simulink model "DSTATCOM"  (R2023b)
settings: Solver=ode5  StartTime=0.0  StopTime=1  FixedStep=50e-8  RelTol=1e-3
InitFcn:
  | v= 400
  | p= 2500
  | q=1500
  | s=2915.47
undefined symbols (not defined in the file): DiscIntNeverNeededParam
libraries: spsThreePhaseVIMeasurementLib x11, spsThreePhaseSeriesRLCBranchLib x9, spsThreePhaseSeriesRLCLoadLib x8, spsSeriesRLCBranchLib x6, spsSecondOrderFilterLib x4, slpidlib x4, spsGroundLib x3, spsLinearTransformerLib x3, spsRMSLib x3, spsUniversalBridgeLib x2, spsabctodq0Lib x2, spsPWMGenerator2LevelLib x2
(part 1 of 2)
settings Model: Creator=prabh  LastModifiedBy=Sandesh

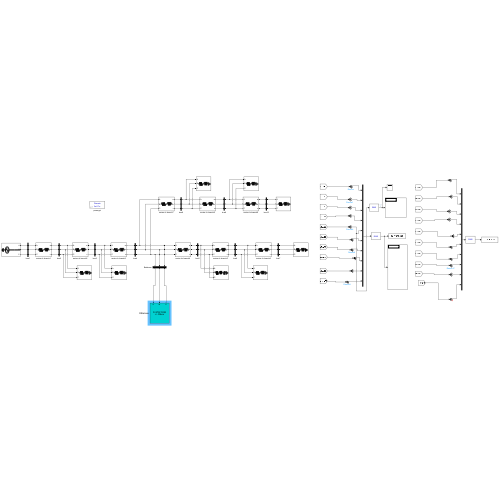
[thumbnail: Simulink's stored preview of the top-level diagram]
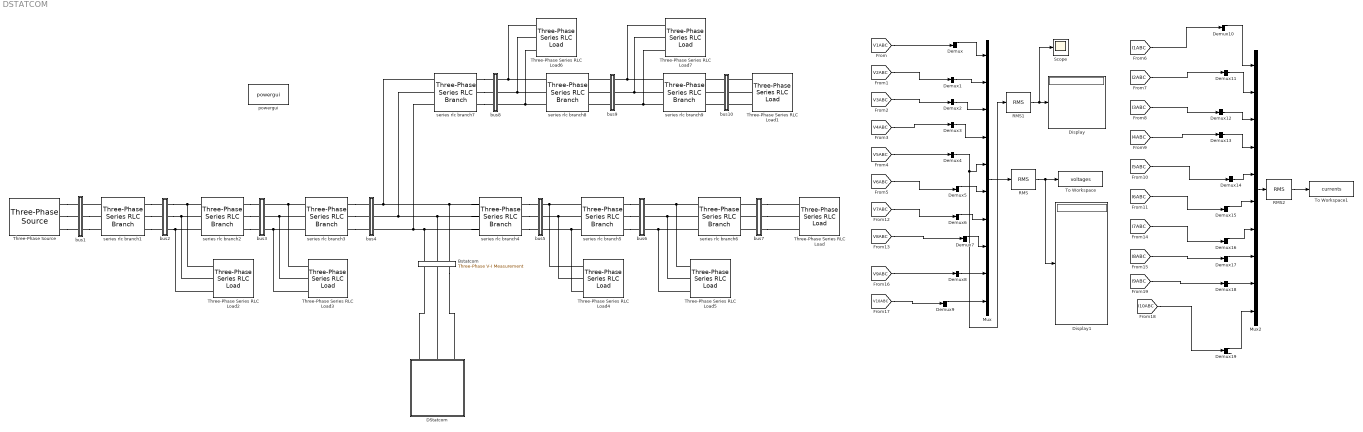
== system DSTATCOM ==
  Bstatcom : spsThreePhaseVIMeasurementLib/Three-Phase V-I Measurement  VoltageMeasurement=phase-to-ground  SetLabelV=on  LabelV=Vabc_Bstatcom  Vpu=on  VpuLL=off  CurrentMeasurement=yes  SetLabelI=on  LabelI=Iabc_Bstatcom  Ipu=on  Pbase=3e3  Vbase=400  OutputType=Magnitude  PhasorSimulation=off  PSBequivalent=0
  DStatcom : Subsystem
      mask Display: disp('D-STATCOM\n+/- 3Mvar')
  Demux{,1..19} (20 alike) : Demux  Outputs=3
  Display : Display
  Display1 : Display
  Mux : Mux  Inputs=10
  Mux2 : Mux  Inputs=10
  RMS : spsRMSLib/RMS  TrueRMS=on  Freq=50  RMSInit=0  Ts=0
  RMS1 : spsRMSLib/RMS  TrueRMS=on  Freq=50  RMSInit=0  Ts=0
  RMS2 : spsRMSLib/RMS  TrueRMS=on  Freq=50  RMSInit=0  Ts=0
  Scope : Scope
  Three-Phase Series RLC Load{,1..3,5..7} (7 alike) : spsThreePhaseSeriesRLCLoadLib/Three-Phase Series RLC Load  LConnTagsString=A|B|C  Configuration=Y (grounded)  NominalVoltage=v  Vabc=[1e3 1e3 1e3]  Vabcp=[1e3 1e3 1e3]  NominalFrequency=50  UnbalancedPower=off  ActivePower=p  InductivePower=q  CapacitivePower=0  Pabc=[10e3 9e3 11e3]  QLabc=[100 90 110]  QCabc=[100 90 110]  Pabcp=[10e3 9e3 11e3]  QLabcp=[100 90 110]  QCabcp=[100 90 110]  Measurements=None  LoadType=constant PQ
  Three-Phase Series RLC Load4 : spsThreePhaseSeriesRLCLoadLib/Three-Phase Series RLC Load  LConnTagsString=A|B|C  Configuration=Y (grounded)  NominalVoltage=v  Vabc=[1e3 1e3 1e3]  Vabcp=[1e3 1e3 1e3]  NominalFrequency=50  UnbalancedPower=off  ActivePower=p  InductivePower=q  CapacitivePower=q  Pabc=[10e3 9e3 11e3]  QLabc=[100 90 110]  QCabc=[100 90 110]  Pabcp=[10e3 9e3 11e3]  QLabcp=[100 90 110]  QCabcp=[100 90 110]  Measurements=None  LoadType=constant PQ
  Three-Phase Source : spsThreePhaseSourceLib/Three-Phase Source  InternalConnection=Yg  VoltagePhases=off  Voltage=400  PhaseAngle=0  Voltage_phases=[25e3 25e3 25e3]/sqrt(3)  PhaseAngles_phases=[0 -120 +120]  Frequency=50  NonIdealSource=off  SpecifyImpedance=off  Resistance=0.8929  Inductance=16.58e-3  ShortCircuitLevel=100e6  BaseVoltage=25e3  XRratio=7  BusType=swing  Pref=10e3  Qref=0  Prefabc=[10e3, 10e3, 10e3]  Qrefabc=[0, 0, 0]  Qmin=-inf  Qmax=inf
  To Workspace : ToWorkspace  VariableName=voltages  SampleTime=-1
      settings: MaxDataPoints=1
  To Workspace1 : ToWorkspace  VariableName=currents  SampleTime=-1
      settings: MaxDataPoints=1
  bus1 : Subsystem
  bus10 : Subsystem
  bus2 : Subsystem
  bus3 : Subsystem
  bus4 : Subsystem
  bus5 : Subsystem
  bus6 : Subsystem
  bus7 : Subsystem
  bus8 : Subsystem
  bus9 : Subsystem
  powergui : sps_lib/powergui  Priority=1  SimulationMode=Discrete  SampleTime=50e-8  frequency=60  Iterations=50  frequencyindice=50  Pbase=100e6  ErrMax=1e-4  UnitsV=kV  UnitsW=MW  buscounter=0  FunctionMessages=off  echomessages=off  EnableUseOfTLC=off  CurrentSourceSwitches=off  DisableSnubberDevices=off  DisableRonSwitches=off  DisableVfSwitches=off  DisplayEquations=off  AutomaticDiscreteSolvers=off  SolverType=Tustin/Backward Euler (TBE)  Interpol=off  ExternalGateDelay=off  methode=off  Ts=100  x0status=blocks  SPID=on  SwTol=0  HookPort=off  NonlinearTolerance=1e-4  nMaxIteration=100  ContinueOnMaxIteration=off  RestoreLinks=warning  ResistiveCurrentMeasurement=off  Frange=[0:2:500]  Ylog=off  Xlog=on  ShowGrid=off  save=off  variable=ZData  structure=0  ZoomFFT=off  StartTime=0.0  cycles=1  DisplayStyle=1  fundamental=60  FreqAxis=off  MaxFrequency=1000  frequencyindicesteady=1  RmsSteady=1  display=off
  series rlc branch1 : spsThreePhaseSeriesRLCBranchLib/Three-Phase Series RLC Branch  LConnTagsString=A|B|C  RConnTagsString=A|B|C  BranchType=RL  Resistance=0.12  Inductance=0.00027  Capacitance=0  Measurements=None
  series rlc branch2 : spsThreePhaseSeriesRLCBranchLib/Three-Phase Series RLC Branch  LConnTagsString=A|B|C  RConnTagsString=A|B|C  BranchType=RL  Resistance=.78  Inductance=.00177  Capacitance=0  Measurements=None
  series rlc branch3 : spsThreePhaseSeriesRLCBranchLib/Three-Phase Series RLC Branch  LConnTagsString=A|B|C  RConnTagsString=A|B|C  BranchType=RL  Resistance=.96  Inductance=.00218  Capacitance=0  Measurements=None
  series rlc branch4 : spsThreePhaseSeriesRLCBranchLib/Three-Phase Series RLC Branch  LConnTagsString=A|B|C  RConnTagsString=A|B|C  BranchType=RL  Resistance=.96  Inductance=.00218  Capacitance=0  Measurements=None
  series rlc branch5 : spsThreePhaseSeriesRLCBranchLib/Three-Phase Series RLC Branch  LConnTagsString=A|B|C  RConnTagsString=A|B|C  BranchType=RL  Resistance=.36  Inductance=.000821  Capacitance=0  Measurements=None
  series rlc branch6 : spsThreePhaseSeriesRLCBranchLib/Three-Phase Series RLC Branch  LConnTagsString=A|B|C  RConnTagsString=A|B|C  BranchType=RL  Resistance=.3  Inductance=.00068  Capacitance=0  Measurements=None
  series rlc branch7 : spsThreePhaseSeriesRLCBranchLib/Three-Phase Series RLC Branch  LConnTagsString=A|B|C  RConnTagsString=A|B|C  BranchType=RL  Resistance=.18  Inductance=.00041  Capacitance=0  Measurements=None
  series rlc branch8 : spsThreePhaseSeriesRLCBranchLib/Three-Phase Series RLC Branch  LConnTagsString=A|B|C  RConnTagsString=A|B|C  BranchType=RL  Resistance=.12  Inductance=.00027  Capacitance=0  Measurements=None
  series rlc branch9 : spsThreePhaseSeriesRLCBranchLib/Three-Phase Series RLC Branch  LConnTagsString=A|B|C  RConnTagsString=A|B|C  BranchType=RL  Resistance=.6  Inductance=.00136  Capacitance=0  Measurements=None
  wires:
  Mux/1 -> RMS/1
  [V1ABC] -> Demux/1
  Demux/1 -> Mux/1
  [V10ABC] -> Demux9/1
  [V9ABC] -> Demux8/1
  [V8ABC] -> Demux7/1
  [V7ABC] -> Demux6/1
  [V6ABC] -> Demux5/1
  [V5ABC] -> Demux4/1
  [V4ABC] -> Demux3/1
  [V3ABC] -> Demux2/1
  [V2ABC] -> Demux1/1
  Demux1/2 -> Mux/2
  Demux2/2 -> Mux/3
  Demux3/2 -> Mux/4
  Demux4/2 -> RMS1/1, Mux/5
  Demux5/1 -> Mux/6
  Demux6/1 -> Mux/7
  Demux7/1 -> Mux/8
  Demux8/2 -> Mux/9
  Demux9/1 -> Mux/10
  [I3ABC] -> Demux12/1
  Demux19/3 -> ?
  [I8ABC] -> Demux17/1
  [I9ABC] -> Demux18/1
  [I10ABC] -> Demux19/1
  [I4ABC] -> Demux13/1
  Demux11/2 -> Mux2/2
  Demux12/2 -> Mux2/3
  Demux18/2 -> Mux2/9
  Demux19/1 -> Mux2/10
  [I6ABC] -> Demux15/1
  [I7ABC] -> Demux16/1
  [I1ABC] -> Demux10/1
  Demux10/1 -> Mux2/1
  Demux13/2 -> Mux2/4
  Demux16/1 -> Mux2/7
  Demux15/1 -> Mux2/6
  Demux14/2 -> Mux2/5
  [I5ABC] -> Demux14/1
  Mux2/1 -> RMS2/1
  [I2ABC] -> Demux11/1
  Demux17/1 -> Mux2/8
  RMS/1 -> Display1/1, To Workspace/1
  RMS2/1 -> To Workspace1/1
  RMS1/1 -> Scope/1, Display/1
  connections:
  series rlc branch1/LConn1 -- bus1/RConn1
  bus1/RConn2 -- series rlc branch1/LConn2
  bus1/RConn3 -- series rlc branch1/LConn3
  Three-Phase Source/RConn2 -- bus1/LConn2
  Three-Phase Source/RConn1 -- bus1/LConn1
  Three-Phase Source/RConn3 -- bus1/LConn3
  series rlc branch1/RConn2 -- bus2/LConn2
  series rlc branch1/RConn1 -- bus2/LConn1
  series rlc branch1/RConn3 -- bus2/LConn3
  series rlc branch2/RConn2 -- bus3/LConn2
  series rlc branch3/LConn2 -- Three-Phase Series RLC Load3/LConn2 -- bus3/RConn2
  bus2/RConn1 -- Three-Phase Series RLC Load2/LConn1 -- series rlc branch2/LConn1
  series rlc branch2/RConn1 -- bus3/LConn1
  series rlc branch2/RConn3 -- bus3/LConn3
  series rlc branch3/LConn1 -- Three-Phase Series RLC Load3/LConn1 -- bus3/RConn1
  bus2/RConn2 -- Three-Phase Series RLC Load2/LConn2 -- series rlc branch2/LConn2
  bus2/RConn3 -- Three-Phase Series RLC Load2/LConn3 -- series rlc branch2/LConn3
  series rlc branch3/LConn3 -- Three-Phase Series RLC Load3/LConn3 -- bus3/RConn3
  series rlc branch3/RConn2 -- bus4/LConn2
  series rlc branch4/LConn2 -- Bstatcom/LConn2 -- bus4/RConn2 -- series rlc branch7/LConn2
  series rlc branch3/RConn1 -- bus4/LConn1
  series rlc branch3/RConn3 -- bus4/LConn3
  series rlc branch4/LConn1 -- Bstatcom/LConn3 -- series rlc branch7/LConn1 -- bus4/RConn1
  series rlc branch4/LConn3 -- Bstatcom/LConn1 -- bus4/RConn3 -- series rlc branch7/LConn3
  series rlc branch4/RConn2 -- bus5/LConn2
  series rlc branch5/LConn2 -- Three-Phase Series RLC Load4/LConn2 -- bus5/RConn2
  series rlc branch4/RConn1 -- bus5/LConn1
  series rlc branch4/RConn3 -- bus5/LConn3
  series rlc branch5/LConn1 -- Three-Phase Series RLC Load4/LConn1 -- bus5/RConn1
  series rlc branch5/LConn3 -- bus5/RConn3 -- Three-Phase Series RLC Load4/LConn3
  series rlc branch5/RConn2 -- bus6/LConn2
  series rlc branch6/LConn2 -- Three-Phase Series RLC Load5/LConn2 -- bus6/RConn2
  series rlc branch5/RConn1 -- bus6/LConn1
  series rlc branch5/RConn3 -- bus6/LConn3
  series rlc branch6/LConn1 -- Three-Phase Series RLC Load5/LConn1 -- bus6/RConn1
  series rlc branch6/LConn3 -- Three-Phase Series RLC Load5/LConn3 -- bus6/RConn3
  series rlc branch8/LConn3 -- Three-Phase Series RLC Load6/LConn3 -- bus8/RConn3
  series rlc branch8/LConn2 -- Three-Phase Series RLC Load6/LConn2 -- bus8/RConn2
  series rlc branch8/LConn1 -- Three-Phase Series RLC Load6/LConn1 -- bus8/RConn1
  series rlc branch7/RConn1 -- bus8/LConn1
  series rlc branch7/RConn2 -- bus8/LConn2
  series rlc branch7/RConn3 -- bus8/LConn3
  bus7/LConn1 -- series rlc branch6/RConn1
  bus7/LConn2 -- series rlc branch6/RConn2
  bus7/LConn3 -- series rlc branch6/RConn3
  bus7/RConn1 -- Three-Phase Series RLC Load/LConn1
  bus7/RConn2 -- Three-Phase Series RLC Load/LConn2
  bus7/RConn3 -- Three-Phase Series RLC Load/LConn3
  bus9/LConn1 -- series rlc branch8/RConn1
  bus9/LConn2 -- series rlc branch8/RConn2
  bus9/LConn3 -- series rlc branch8/RConn3
  series rlc branch9/LConn1 -- Three-Phase Series RLC Load7/LConn1 -- bus9/RConn1
  series rlc branch9/LConn2 -- Three-Phase Series RLC Load7/LConn2 -- bus9/RConn2
  series rlc branch9/LConn3 -- Three-Phase Series RLC Load7/LConn3 -- bus9/RConn3
  bus10/LConn1 -- series rlc branch9/RConn1
  bus10/LConn2 -- series rlc branch9/RConn2
  bus10/LConn3 -- series rlc branch9/RConn3
  Three-Phase Series RLC Load1/LConn1 -- bus10/RConn1
  Three-Phase Series RLC Load1/LConn2 -- bus10/RConn2
  Three-Phase Series RLC Load1/LConn3 -- bus10/RConn3
  DStatcom/RConn1 -- Bstatcom/RConn1
  Bstatcom/RConn3 -- DStatcom/RConn3
  DStatcom/RConn2 -- Bstatcom/RConn2

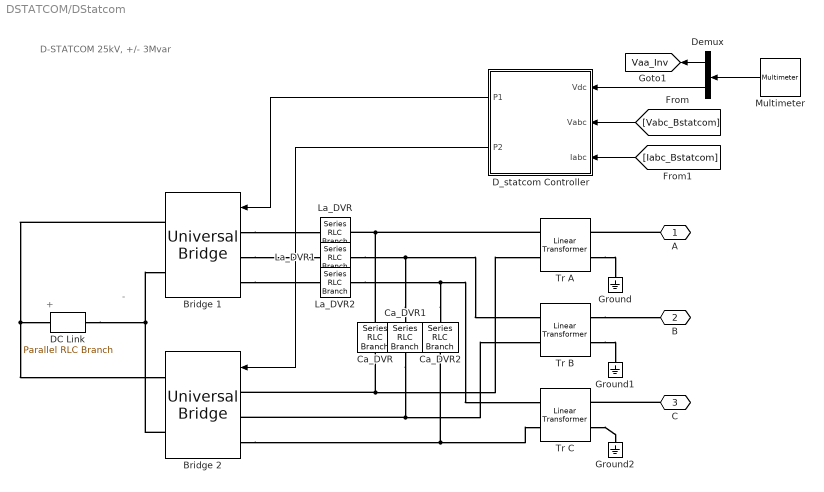
== system DSTATCOM/DStatcom ==
  note: +
  note: -
  note: D-STATCOM
      | 25kV, +/- 3Mvar
  "Bridge 1 " : spsUniversalBridgeLib/Universal Bridge  Arms=3  SnubberResistance=1e5  SnubberCapacitance=inf  Device=IGBT / Diodes  Ron=1e-3  Lon=0  ForwardVoltages="[  2  0.8  ]"  ForwardVoltage=.8  GTOparameters=[ 10e-6 , 20e-6 ]  IGBTparameters=[ 0 0]  Measurements=Device voltages  Measurements_2=None  converterType=Rectifier
      settings: AttributesFormatString=\n
  Bridge 2 : spsUniversalBridgeLib/Universal Bridge  Arms=3  SnubberResistance=1e5  SnubberCapacitance=inf  Device=IGBT / Diodes  Ron=1e-3  Lon=0  ForwardVoltages="[  2  0.8  ]"  ForwardVoltage=.8  GTOparameters=[ 10e-6 , 20e-6 ]  IGBTparameters=[ 0 0]  Measurements=Device voltages  Measurements_2=None  converterType=Rectifier
      settings: AttributesFormatString=\n
  Ca_DVR : spsSeriesRLCBranchLib/Series RLC Branch  LConnTagsString=__new0  RConnTagsString=__new0  BranchType=RC  Resistance=100e-6*(2*pi*60)/40  Inductance=1.0  SetiL0=off  InitialCurrent=0  Capacitance=100e-6  Setx0=off  InitialVoltage=0  Measurements=None
  Ca_DVR1 : spsSeriesRLCBranchLib/Series RLC Branch  LConnTagsString=__new0  RConnTagsString=__new0  BranchType=RC  Resistance=100e-6*(2*pi*60)/40  Inductance=1.0  SetiL0=off  InitialCurrent=0  Capacitance=100e-6  Setx0=off  InitialVoltage=0  Measurements=None
  Ca_DVR2 : spsSeriesRLCBranchLib/Series RLC Branch  LConnTagsString=__new0  RConnTagsString=__new0  BranchType=RC  Resistance=100e-6*(2*pi*60)/40  Inductance=1.0  SetiL0=off  InitialCurrent=0  Capacitance=100e-6  Setx0=off  InitialVoltage=0  Measurements=None
  DC Link : spsParallelRLCBranchLib/Parallel RLC Branch  LConnTagsString=a  RConnTagsString=__new0  BranchType=C  Resistance=1.0  Inductance=1.0  SetiL0=off  InitialCurrent=0  Capacitance=5000e-6  Setx0=on  InitialVoltage=0  Measurements=Branch voltage
  D_statcom Controller : Subsystem  mask(D-STATCOM Controller){ModeOper=Voltage regulation, Vac_Ref=1.0, Qref=0, Vdc_Ref=2400, Par_VacReg=[0.55 2500], Par_VdcReg=[0.001 0.15], Par_IReg=[0.8 200 0], Ts=50e-8}
      mask prompts: ModeOper "Mode of operation:"; Vac_Ref "AC voltage setpoint Vref (pu):"; Qref "Manual mode: Qref (Reactive power in pu):"; Vdc_Ref "DC Voltage setpoint (Volts)"; Par_VacReg "Vac Regulator Gains: [ Kp  Ki ]"; Par_VdcReg "Vdc Regulator Gains: [ Kp  Ki ]"; Par_IReg "Current Regulators Gain: [ Kp Ki Kd ]"; Ts "Sample time (s)"
      mask init:
      | Kp_I=Par_IReg(1);
      | Ki_I=Par_IReg(2);
      | Kd_I=Par_IReg(3);
      | Kp_Vdc=Par_VdcReg(1);
      | Ki_Vdc=Par_VdcReg(2);
      | Kp_Vac=Par_VacReg(1);
      | Ki_Vac=Par_VacReg(2);
      mask TypeOptions ModeOper: Voltage regulation | Q regulation
  Demux : Demux  Outputs=[2 1 ]
      settings: DisplayOption=none
  Ground : spsGroundLib/Ground  LConnTagsString=a
  Ground1 : spsGroundLib/Ground  LConnTagsString=a
  Ground2 : spsGroundLib/Ground  LConnTagsString=a
  La_DVR : spsSeriesRLCBranchLib/Series RLC Branch  LConnTagsString=__new0  RConnTagsString=__new0  BranchType=L  Resistance=1.0  Inductance=800e-6  SetiL0=off  InitialCurrent=0  Capacitance=1.0  Setx0=off  InitialVoltage=0  Measurements=None
  La_DVR1 : spsSeriesRLCBranchLib/Series RLC Branch  LConnTagsString=__new0  RConnTagsString=__new0  BranchType=L  Resistance=1.0  Inductance=800e-6  SetiL0=off  InitialCurrent=0  Capacitance=1.0  Setx0=off  InitialVoltage=0  Measurements=None
  La_DVR2 : spsSeriesRLCBranchLib/Series RLC Branch  LConnTagsString=__new0  RConnTagsString=__new0  BranchType=L  Resistance=1.0  Inductance=800e-6  SetiL0=off  InitialCurrent=0  Capacitance=1.0  Setx0=off  InitialVoltage=0  Measurements=None
  Multimeter : spsMultimeterLib/Multimeter  Tag=PoWeRsYsTeMmEaSuReMeNt  L=13  sel=[3 9 1]  yselected={}  Gain=[1 1 1]  OutputType=Magnitude  PlotAtSimulationStop=off  PhasorSimulation=off
      settings: AttributesFormatString=\n
  Tr A : spsLinearTransformerLib/Linear Transformer  UNITS=pu  NominalPower=[3e6/3 60]  winding1=[1250 0.03/30 0.03]  winding2=[25e3/sqrt(3) 0.03/30 0.03]  ThreeWindings=off  winding3=[60e3 0.005 0.02]  RmLm=[200 200]  Measurements=None  DataType=off
  Tr B : spsLinearTransformerLib/Linear Transformer  UNITS=pu  NominalPower=[3e6/3 60]  winding1=[1250 0.03/30 0.03]  winding2=[25e3/sqrt(3) 0.03/30 0.03]  ThreeWindings=off  winding3=[60e3 0.005 0.02]  RmLm=[200 200]  Measurements=None  DataType=off
  Tr C : spsLinearTransformerLib/Linear Transformer  UNITS=pu  NominalPower=[3e6/3 60]  winding1=[1250 0.03/30 0.03]  winding2=[25e3/sqrt(3) 0.03/30 0.03]  ThreeWindings=off  winding3=[60e3 0.005 0.02]  RmLm=[200 200]  Measurements=None  DataType=off
  A : PMIOPort  Side=Right
  B : PMIOPort  Port=2  Side=Right
  C : PMIOPort  Port=3  Side=Right
  tag scope: Vaa_Inv=global
  wires:
  Multimeter/1 -> Demux/1
  Demux/2 -> D_statcom Controller/1(Vdc)
  Demux/1 -> [Vaa_Inv]
  [Vabc_Bstatcom] -> D_statcom Controller/2(Vabc)
  [Iabc_Bstatcom] -> D_statcom Controller/3(Iabc)
  D_statcom Controller/1(P1) -> "Bridge 1 "/1
  D_statcom Controller/2(P2) -> Bridge 2/1
  connections:
  "Bridge 1 "/LConn1 -- La_DVR/LConn1
  "Bridge 1 "/LConn2 -- La_DVR1/LConn1
  "Bridge 1 "/LConn3 -- La_DVR2/LConn1
  Bridge 2/LConn2 -- Tr B/LConn2 -- Ca_DVR1/LConn1
  Bridge 2/LConn3 -- Tr C/LConn2 -- Ca_DVR2/LConn1
  Ca_DVR1/RConn1 -- La_DVR1/RConn1 -- Tr B/LConn1
  Ca_DVR2/RConn1 -- La_DVR2/RConn1 -- Tr C/LConn1
  Tr A/LConn1 -- La_DVR/RConn1 -- Ca_DVR/RConn1
  Tr C/RConn2 -- Ground2/LConn1
  Tr B/RConn2 -- Ground1/LConn1
  Tr A/RConn2 -- Ground/LConn1
  A/RConn1 -- Tr A/RConn1
  Tr B/RConn1 -- B/RConn1
  C/RConn1 -- Tr C/RConn1
  "Bridge 1 "/RConn1 -- Bridge 2/RConn1 -- DC Link/LConn1
  Bridge 2/RConn2 -- "Bridge 1 "/RConn2 -- DC Link/RConn1
  Bridge 2/LConn1 -- Tr A/LConn2 -- Ca_DVR/LConn1

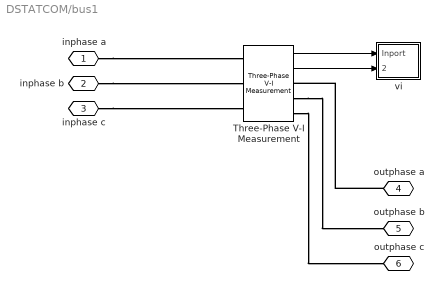
== system DSTATCOM/bus1 ==
  Three-Phase V-I Measurement : spsThreePhaseVIMeasurementLib/Three-Phase V-I Measurement  VoltageMeasurement=phase-to-ground  SetLabelV=off  LabelV=Vabc  Vpu=off  VpuLL=off  CurrentMeasurement=yes  SetLabelI=off  LabelI=Iabc  Ipu=off  Pbase=100e6  Vbase=500e3  OutputType=Complex  PhasorSimulation=off  PSBequivalent=0
  vi : Subsystem
  inphase a : PMIOPort  Side=Left
  inphase b : PMIOPort  Port=2  Side=Left
  inphase c : PMIOPort  Port=3  Side=Left
  outphase a : PMIOPort  Port=4  Side=Right
  outphase b : PMIOPort  Port=5  Side=Right
  outphase c : PMIOPort  Port=6  Side=Right
  wires:
  Three-Phase V-I Measurement/1 -> vi/1(Inport)
  Three-Phase V-I Measurement/2 -> vi/2(Inport1)
  connections:
  inphase a/RConn1 -- Three-Phase V-I Measurement/LConn1
  inphase b/RConn1 -- Three-Phase V-I Measurement/LConn2
  inphase c/RConn1 -- Three-Phase V-I Measurement/LConn3
  outphase a/RConn1 -- Three-Phase V-I Measurement/RConn1
  Three-Phase V-I Measurement/RConn2 -- outphase b/RConn1
  Three-Phase V-I Measurement/RConn3 -- outphase c/RConn1

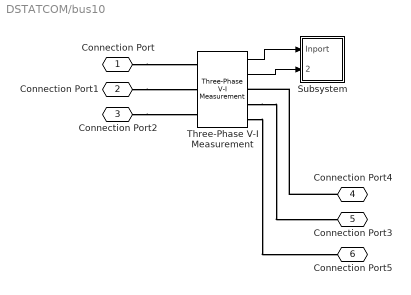
== system DSTATCOM/bus10 ==
  Subsystem : Subsystem
  Three-Phase V-I Measurement : spsThreePhaseVIMeasurementLib/Three-Phase V-I Measurement  VoltageMeasurement=phase-to-ground  SetLabelV=off  LabelV=Vabc  Vpu=off  VpuLL=off  CurrentMeasurement=yes  SetLabelI=off  LabelI=Iabc  Ipu=off  Pbase=100e6  Vbase=500e3  OutputType=Complex  PhasorSimulation=off  PSBequivalent=0
  Connection Port : PMIOPort  Side=Left
  Connection Port1 : PMIOPort  Port=2  Side=Left
  Connection Port2 : PMIOPort  Port=3  Side=Left
  Connection Port4 : PMIOPort  Port=4  Side=Right
  Connection Port3 : PMIOPort  Port=5  Side=Right
  Connection Port5 : PMIOPort  Port=6  Side=Right
  wires:
  Three-Phase V-I Measurement/1 -> Subsystem/1(Inport)
  Three-Phase V-I Measurement/2 -> Subsystem/2(Inport1)
  connections:
  Connection Port/RConn1 -- Three-Phase V-I Measurement/LConn1
  Connection Port1/RConn1 -- Three-Phase V-I Measurement/LConn2
  Connection Port2/RConn1 -- Three-Phase V-I Measurement/LConn3
  Connection Port4/RConn1 -- Three-Phase V-I Measurement/RConn1
  Three-Phase V-I Measurement/RConn2 -- Connection Port3/RConn1
  Three-Phase V-I Measurement/RConn3 -- Connection Port5/RConn1

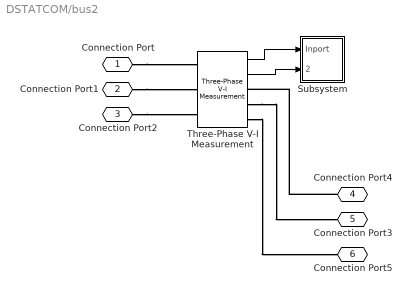
== system DSTATCOM/bus2 ==
  Subsystem : Subsystem
  Three-Phase V-I Measurement : spsThreePhaseVIMeasurementLib/Three-Phase V-I Measurement  VoltageMeasurement=phase-to-ground  SetLabelV=off  LabelV=Vabc  Vpu=off  VpuLL=off  CurrentMeasurement=yes  SetLabelI=off  LabelI=Iabc  Ipu=off  Pbase=100e6  Vbase=500e3  OutputType=Complex  PhasorSimulation=off  PSBequivalent=0
  Connection Port : PMIOPort  Side=Left
  Connection Port1 : PMIOPort  Port=2  Side=Left
  Connection Port2 : PMIOPort  Port=3  Side=Left
  Connection Port4 : PMIOPort  Port=4  Side=Right
  Connection Port3 : PMIOPort  Port=5  Side=Right
  Connection Port5 : PMIOPort  Port=6  Side=Right
  wires:
  Three-Phase V-I Measurement/1 -> Subsystem/1(Inport)
  Three-Phase V-I Measurement/2 -> Subsystem/2(Inport1)
  connections:
  Connection Port/RConn1 -- Three-Phase V-I Measurement/LConn1
  Connection Port1/RConn1 -- Three-Phase V-I Measurement/LConn2
  Connection Port2/RConn1 -- Three-Phase V-I Measurement/LConn3
  Connection Port4/RConn1 -- Three-Phase V-I Measurement/RConn1
  Three-Phase V-I Measurement/RConn2 -- Connection Port3/RConn1
  Three-Phase V-I Measurement/RConn3 -- Connection Port5/RConn1

== system DSTATCOM/bus3 ==
  Subsystem : Subsystem
  Three-Phase V-I Measurement : spsThreePhaseVIMeasurementLib/Three-Phase V-I Measurement  VoltageMeasurement=phase-to-ground  SetLabelV=off  LabelV=Vabc  Vpu=off  VpuLL=off  CurrentMeasurement=yes  SetLabelI=off  LabelI=Iabc  Ipu=off  Pbase=100e6  Vbase=500e3  OutputType=Complex  PhasorSimulation=off  PSBequivalent=0
  Connection Port : PMIOPort  Side=Left
  Connection Port1 : PMIOPort  Port=2  Side=Left
  Connection Port2 : PMIOPort  Port=3  Side=Left
  Connection Port4 : PMIOPort  Port=4  Side=Right
  Connection Port3 : PMIOPort  Port=5  Side=Right
  Connection Port5 : PMIOPort  Port=6  Side=Right
  wires:
  Three-Phase V-I Measurement/1 -> Subsystem/1(Inport)
  Three-Phase V-I Measurement/2 -> Subsystem/2(Inport1)
  connections:
  Connection Port/RConn1 -- Three-Phase V-I Measurement/LConn1
  Connection Port1/RConn1 -- Three-Phase V-I Measurement/LConn2
  Connection Port2/RConn1 -- Three-Phase V-I Measurement/LConn3
  Connection Port4/RConn1 -- Three-Phase V-I Measurement/RConn1
  Three-Phase V-I Measurement/RConn2 -- Connection Port3/RConn1
  Three-Phase V-I Measurement/RConn3 -- Connection Port5/RConn1

== system DSTATCOM/bus4 ==
  Subsystem : Subsystem
  Three-Phase V-I Measurement : spsThreePhaseVIMeasurementLib/Three-Phase V-I Measurement  VoltageMeasurement=phase-to-ground  SetLabelV=off  LabelV=Vabc  Vpu=off  VpuLL=off  CurrentMeasurement=yes  SetLabelI=off  LabelI=Iabc  Ipu=off  Pbase=100e6  Vbase=500e3  OutputType=Complex  PhasorSimulation=off  PSBequivalent=0
  Connection Port : PMIOPort  Side=Left
  Connection Port1 : PMIOPort  Port=2  Side=Left
  Connection Port2 : PMIOPort  Port=3  Side=Left
  Connection Port4 : PMIOPort  Port=4  Side=Right
  Connection Port3 : PMIOPort  Port=5  Side=Right
  Connection Port5 : PMIOPort  Port=6  Side=Right
  wires:
  Three-Phase V-I Measurement/1 -> Subsystem/1(Inport)
  Three-Phase V-I Measurement/2 -> Subsystem/2(Inport1)
  connections:
  Connection Port/RConn1 -- Three-Phase V-I Measurement/LConn1
  Connection Port1/RConn1 -- Three-Phase V-I Measurement/LConn2
  Connection Port2/RConn1 -- Three-Phase V-I Measurement/LConn3
  Connection Port4/RConn1 -- Three-Phase V-I Measurement/RConn1
  Three-Phase V-I Measurement/RConn2 -- Connection Port3/RConn1
  Three-Phase V-I Measurement/RConn3 -- Connection Port5/RConn1

== system DSTATCOM/bus5 ==
  Subsystem : Subsystem
  Three-Phase V-I Measurement : spsThreePhaseVIMeasurementLib/Three-Phase V-I Measurement  VoltageMeasurement=phase-to-ground  SetLabelV=off  LabelV=Vabc  Vpu=off  VpuLL=off  CurrentMeasurement=yes  SetLabelI=off  LabelI=Iabc  Ipu=off  Pbase=100e6  Vbase=500e3  OutputType=Complex  PhasorSimulation=off  PSBequivalent=0
  Connection Port : PMIOPort  Side=Left
  Connection Port1 : PMIOPort  Port=2  Side=Left
  Connection Port2 : PMIOPort  Port=3  Side=Left
  Connection Port4 : PMIOPort  Port=4  Side=Right
  Connection Port3 : PMIOPort  Port=5  Side=Right
  Connection Port5 : PMIOPort  Port=6  Side=Right
  wires:
  Three-Phase V-I Measurement/1 -> Subsystem/1(Inport)
  Three-Phase V-I Measurement/2 -> Subsystem/2(Inport1)
  connections:
  Connection Port/RConn1 -- Three-Phase V-I Measurement/LConn1
  Connection Port1/RConn1 -- Three-Phase V-I Measurement/LConn2
  Connection Port2/RConn1 -- Three-Phase V-I Measurement/LConn3
  Connection Port4/RConn1 -- Three-Phase V-I Measurement/RConn1
  Three-Phase V-I Measurement/RConn2 -- Connection Port3/RConn1
  Three-Phase V-I Measurement/RConn3 -- Connection Port5/RConn1

== system DSTATCOM/bus6 ==
  Subsystem : Subsystem
  Three-Phase V-I Measurement : spsThreePhaseVIMeasurementLib/Three-Phase V-I Measurement  VoltageMeasurement=phase-to-ground  SetLabelV=off  LabelV=Vabc  Vpu=off  VpuLL=off  CurrentMeasurement=yes  SetLabelI=off  LabelI=Iabc  Ipu=off  Pbase=100e6  Vbase=500e3  OutputType=Complex  PhasorSimulation=off  PSBequivalent=0
  Connection Port : PMIOPort  Side=Left
  Connection Port1 : PMIOPort  Port=2  Side=Left
  Connection Port2 : PMIOPort  Port=3  Side=Left
  Connection Port4 : PMIOPort  Port=4  Side=Right
  Connection Port3 : PMIOPort  Port=5  Side=Right
  Connection Port5 : PMIOPort  Port=6  Side=Right
  wires:
  Three-Phase V-I Measurement/1 -> Subsystem/1(Inport)
  Three-Phase V-I Measurement/2 -> Subsystem/2(Inport1)
  connections:
  Connection Port/RConn1 -- Three-Phase V-I Measurement/LConn1
  Connection Port1/RConn1 -- Three-Phase V-I Measurement/LConn2
  Connection Port2/RConn1 -- Three-Phase V-I Measurement/LConn3
  Connection Port4/RConn1 -- Three-Phase V-I Measurement/RConn1
  Three-Phase V-I Measurement/RConn2 -- Connection Port3/RConn1
  Three-Phase V-I Measurement/RConn3 -- Connection Port5/RConn1

== system DSTATCOM/bus7 ==
  Subsystem : Subsystem
  Three-Phase V-I Measurement : spsThreePhaseVIMeasurementLib/Three-Phase V-I Measurement  VoltageMeasurement=phase-to-ground  SetLabelV=off  LabelV=Vabc  Vpu=off  VpuLL=off  CurrentMeasurement=yes  SetLabelI=off  LabelI=Iabc  Ipu=off  Pbase=100e6  Vbase=500e3  OutputType=Complex  PhasorSimulation=off  PSBequivalent=0
  Connection Port : PMIOPort  Side=Left
  Connection Port1 : PMIOPort  Port=2  Side=Left
  Connection Port2 : PMIOPort  Port=3  Side=Left
  Connection Port4 : PMIOPort  Port=4  Side=Right
  Connection Port3 : PMIOPort  Port=5  Side=Right
  Connection Port5 : PMIOPort  Port=6  Side=Right
  wires:
  Three-Phase V-I Measurement/1 -> Subsystem/1(Inport)
  Three-Phase V-I Measurement/2 -> Subsystem/2(Inport1)
  connections:
  Connection Port/RConn1 -- Three-Phase V-I Measurement/LConn1
  Connection Port1/RConn1 -- Three-Phase V-I Measurement/LConn2
  Connection Port2/RConn1 -- Three-Phase V-I Measurement/LConn3
  Connection Port4/RConn1 -- Three-Phase V-I Measurement/RConn1
  Three-Phase V-I Measurement/RConn2 -- Connection Port3/RConn1
  Three-Phase V-I Measurement/RConn3 -- Connection Port5/RConn1

== system DSTATCOM/bus8 ==
  Subsystem : Subsystem
  Three-Phase V-I Measurement : spsThreePhaseVIMeasurementLib/Three-Phase V-I Measurement  VoltageMeasurement=phase-to-ground  SetLabelV=off  LabelV=Vabc  Vpu=off  VpuLL=off  CurrentMeasurement=yes  SetLabelI=off  LabelI=Iabc  Ipu=off  Pbase=100e6  Vbase=500e3  OutputType=Complex  PhasorSimulation=off  PSBequivalent=0
  Connection Port : PMIOPort  Side=Left
  Connection Port1 : PMIOPort  Port=2  Side=Left
  Connection Port2 : PMIOPort  Port=3  Side=Left
  Connection Port4 : PMIOPort  Port=4  Side=Right
  Connection Port3 : PMIOPort  Port=5  Side=Right
  Connection Port5 : PMIOPort  Port=6  Side=Right
  wires:
  Three-Phase V-I Measurement/1 -> Subsystem/1(Inport)
  Three-Phase V-I Measurement/2 -> Subsystem/2(Inport1)
  connections:
  Connection Port/RConn1 -- Three-Phase V-I Measurement/LConn1
  Connection Port1/RConn1 -- Three-Phase V-I Measurement/LConn2
  Connection Port2/RConn1 -- Three-Phase V-I Measurement/LConn3
  Connection Port4/RConn1 -- Three-Phase V-I Measurement/RConn1
  Three-Phase V-I Measurement/RConn2 -- Connection Port3/RConn1
  Three-Phase V-I Measurement/RConn3 -- Connection Port5/RConn1

== system DSTATCOM/bus9 ==
  Subsystem : Subsystem
  Three-Phase V-I Measurement : spsThreePhaseVIMeasurementLib/Three-Phase V-I Measurement  VoltageMeasurement=phase-to-ground  SetLabelV=off  LabelV=Vabc  Vpu=off  VpuLL=off  CurrentMeasurement=yes  SetLabelI=off  LabelI=Iabc  Ipu=off  Pbase=100e6  Vbase=500e3  OutputType=Complex  PhasorSimulation=off  PSBequivalent=0
  Connection Port : PMIOPort  Side=Left
  Connection Port1 : PMIOPort  Port=2  Side=Left
  Connection Port2 : PMIOPort  Port=3  Side=Left
  Connection Port4 : PMIOPort  Port=4  Side=Right
  Connection Port3 : PMIOPort  Port=5  Side=Right
  Connection Port5 : PMIOPort  Port=6  Side=Right
  wires:
  Three-Phase V-I Measurement/1 -> Subsystem/1(Inport)
  Three-Phase V-I Measurement/2 -> Subsystem/2(Inport1)
  connections:
  Connection Port/RConn1 -- Three-Phase V-I Measurement/LConn1
  Connection Port1/RConn1 -- Three-Phase V-I Measurement/LConn2
  Connection Port2/RConn1 -- Three-Phase V-I Measurement/LConn3
  Connection Port4/RConn1 -- Three-Phase V-I Measurement/RConn1
  Three-Phase V-I Measurement/RConn2 -- Connection Port3/RConn1
  Three-Phase V-I Measurement/RConn3 -- Connection Port5/RConn1

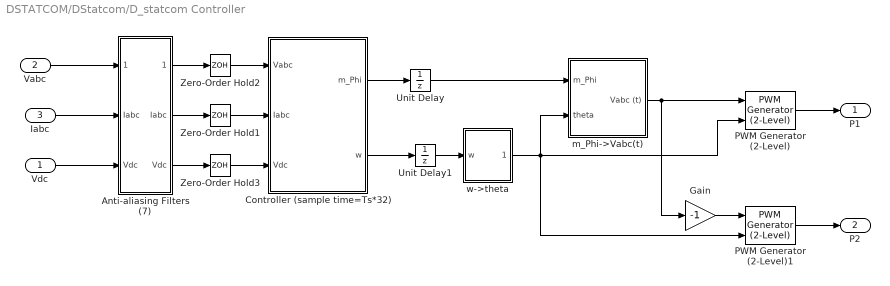
== system DSTATCOM/DStatcom/D_statcom Controller ==
  Vdc : Inport  PortDimensions=1
  Vabc : Inport  Port=2  PortDimensions=3
  Iabc : Inport  Port=3  PortDimensions=3
  Anti-aliasing Filters (7) : Subsystem  mask(Anti-aliasing (2nd order lowpass)){Fc=2000, Ts=50e-8}
      mask prompts: Fc "Cut-off frequency (Hz):"; Ts "Sample time:"
  Controller (sample time=Ts*32) : Subsystem
  Gain : Gain  Gain=-1
  PWM Generator (2-Level) : spsPWMGenerator2LevelLib/PWM Generator (2-Level)  ModulatorType=Three-phase bridge (6 pulses)  ModulatorMode=Synchronized  Fc=27*60  Pc=90  nF=28  MinMax="[ -1  1 ]"  SamplingTechnique=Natural  ModulatingSignals=off  m=0.8  Freq=60  Phase=0  Ts=50e-8  ShowCarrierOutport=off
  PWM Generator (2-Level)1 : spsPWMGenerator2LevelLib/PWM Generator (2-Level)  ModulatorType=Three-phase bridge (6 pulses)  ModulatorMode=Synchronized  Fc=27*60  Pc=90  nF=28  MinMax="[ -1  1 ]"  SamplingTechnique=Natural  ModulatingSignals=off  m=0.8  Freq=60  Phase=0  Ts=50e-8  ShowCarrierOutport=off
  Unit Delay : UnitDelay  SampleTime=50e-8*32  HasFrameUpgradeWarning=on
  Unit Delay1 : UnitDelay  SampleTime=50e-8*32  HasFrameUpgradeWarning=on
  Zero-Order Hold1 : ZeroOrderHold  SampleTime=50e-8*32
  Zero-Order Hold2 : ZeroOrderHold  SampleTime=50e-8*32
  Zero-Order Hold3 : ZeroOrderHold  SampleTime=50e-8*32
  m_Phi->Vabc(t) : Subsystem
  w->theta : Subsystem
  P1 : Outport  VectorParamsAs1DForOutWhenUnconnected=off
  P2 : Outport  Port=2  VectorParamsAs1DForOutWhenUnconnected=off
  wires:
  Gain/1 -> PWM Generator (2-Level)1/1
  PWM Generator (2-Level)1/1 -> P2/1
  PWM Generator (2-Level)/1 -> P1/1
  Anti-aliasing Filters (7)/1(" Vabc") -> Zero-Order Hold2/1
  Anti-aliasing Filters (7)/2(Iabc) -> Zero-Order Hold1/1
  Anti-aliasing Filters (7)/3(" Vdc") -> Zero-Order Hold3/1
  Vabc/1 -> Anti-aliasing Filters (7)/1(Vabc)
  Iabc/1 -> Anti-aliasing Filters (7)/2("Iabc ")
  Vdc/1 -> Anti-aliasing Filters (7)/3("Vdc ")
  Zero-Order Hold2/1 -> Controller (sample time=Ts*32)/1(Vabc)
  Zero-Order Hold1/1 -> Controller (sample time=Ts*32)/2(Iabc)
  Zero-Order Hold3/1 -> Controller (sample time=Ts*32)/3(Vdc)
  Controller (sample time=Ts*32)/1(m_Phi) -> Unit Delay/1
  Unit Delay/1 -> m_Phi->Vabc(t)/1(m_Phi)
  Controller (sample time=Ts*32)/2(w) -> Unit Delay1/1
  Unit Delay1/1 -> w->theta/1(w)
  m_Phi->Vabc(t)/1(Vabc (t)) -> PWM Generator (2-Level)/1, Gain/1
  w->theta/1(theta) -> PWM Generator (2-Level)/2, m_Phi->Vabc(t)/2(theta), PWM Generator (2-Level)1/2

== system DSTATCOM/bus1/vi ==
  Inport : Inport
  Inport1 : Inport  Port=2
  tag scope: I1ABC=global, V1ABC=global
  wires:
  Inport/1 -> [V1ABC]
  Inport1/1 -> [I1ABC]

== system DSTATCOM/bus10/Subsystem ==
  Inport : Inport
  Inport1 : Inport  Port=2
  tag scope: I10ABC=global, V10ABC=global
  wires:
  Inport/1 -> [V10ABC]
  Inport1/1 -> [I10ABC]

== system DSTATCOM/bus2/Subsystem ==
  Inport : Inport
  Inport1 : Inport  Port=2
  tag scope: I2ABC=global, V2ABC=global
  wires:
  Inport/1 -> [V2ABC]
  Inport1/1 -> [I2ABC]

== system DSTATCOM/bus3/Subsystem ==
  Inport : Inport
  Inport1 : Inport  Port=2
  tag scope: I3ABC=global, V3ABC=global
  wires:
  Inport/1 -> [V3ABC]
  Inport1/1 -> [I3ABC]

== system DSTATCOM/bus4/Subsystem ==
  Inport : Inport
  Inport1 : Inport  Port=2
  tag scope: I4ABC=global, V4ABC=global
  wires:
  Inport/1 -> [V4ABC]
  Inport1/1 -> [I4ABC]

== system DSTATCOM/bus5/Subsystem ==
  Inport : Inport
  Inport1 : Inport  Port=2
  tag scope: I5ABC=global, V5ABC=global
  wires:
  Inport/1 -> [V5ABC]
  Inport1/1 -> [I5ABC]

== system DSTATCOM/bus6/Subsystem ==
  Inport : Inport
  Inport1 : Inport  Port=2
  tag scope: I6ABC=global, V6ABC=global
  wires:
  Inport/1 -> [V6ABC]
  Inport1/1 -> [I6ABC]

== system DSTATCOM/bus7/Subsystem ==
  Inport : Inport
  Inport1 : Inport  Port=2
  tag scope: I7ABC=global, V7ABC=global
  wires:
  Inport/1 -> [V7ABC]
  Inport1/1 -> [I7ABC]

== system DSTATCOM/bus8/Subsystem ==
  Inport : Inport
  Inport1 : Inport  Port=2
  tag scope: I8ABC=global, V8ABC=global
  wires:
  Inport/1 -> [V8ABC]
  Inport1/1 -> [I8ABC]

== system DSTATCOM/bus9/Subsystem ==
  Inport : Inport
  Inport1 : Inport  Port=2
  tag scope: I9ABC=global, V9ABC=global
  wires:
  Inport/1 -> [V9ABC]
  Inport1/1 -> [I9ABC]

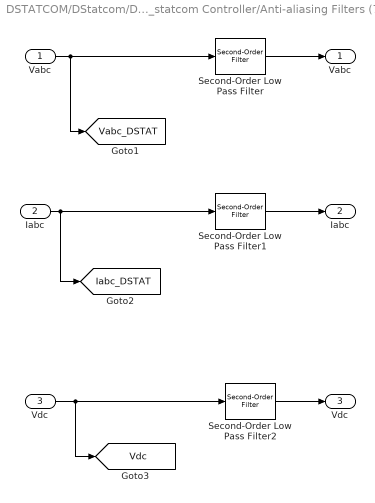
== system DSTATCOM/DStatcom/D_statcom Controller/Anti-aliasing Filters (7) ==
  Vabc : Inport  PortDimensions=3
  "Iabc " : Inport  Port=2  PortDimensions=3
  "Vdc " : Inport  Port=3  PortDimensions=1
  Second-Order Low Pass Filter : spsSecondOrderFilterLib/Second-Order Filter  FilterType=Lowpass  Fo=2000  Zeta=0.707  Ts=50e-8  Initialize=off  Vac_Init="[0,  0,  60]"  Vdc_Init=0  PlotResponse=off  FreqRange=[0, 500, 1]
      settings: AttributesFormatString=f0: %<Fo>
  Second-Order Low Pass Filter1 : spsSecondOrderFilterLib/Second-Order Filter  FilterType=Lowpass  Fo=2000  Zeta=0.707  Ts=50e-8  Initialize=off  Vac_Init="[0,  0,  60]"  Vdc_Init=0  PlotResponse=off  FreqRange=[0, 500, 1]
      settings: AttributesFormatString=f0: %<Fo>
  Second-Order Low Pass Filter2 : spsSecondOrderFilterLib/Second-Order Filter  FilterType=Lowpass  Fo=2000  Zeta=0.707  Ts=50e-8  Initialize=off  Vac_Init="[0,  0,  60]"  Vdc_Init=0  PlotResponse=off  FreqRange=[0, 500, 1]
      settings: AttributesFormatString=f0: %<Fo>
  " Vabc" : Outport  VectorParamsAs1DForOutWhenUnconnected=off
  Iabc : Outport  Port=2  VectorParamsAs1DForOutWhenUnconnected=off
  " Vdc" : Outport  Port=3  VectorParamsAs1DForOutWhenUnconnected=off
  tag scope: Iabc_DSTAT=global, Vabc_DSTAT=global, Vdc=global
  wires:
  Second-Order Low Pass Filter/1 -> " Vabc"/1
  Second-Order Low Pass Filter1/1 -> Iabc/1
  "Iabc "/1 -> [Iabc_DSTAT], Second-Order Low Pass Filter1/1
  Vabc/1 -> [Vabc_DSTAT], Second-Order Low Pass Filter/1
  "Vdc "/1 -> [Vdc], Second-Order Low Pass Filter2/1
  Second-Order Low Pass Filter2/1 -> " Vdc"/1

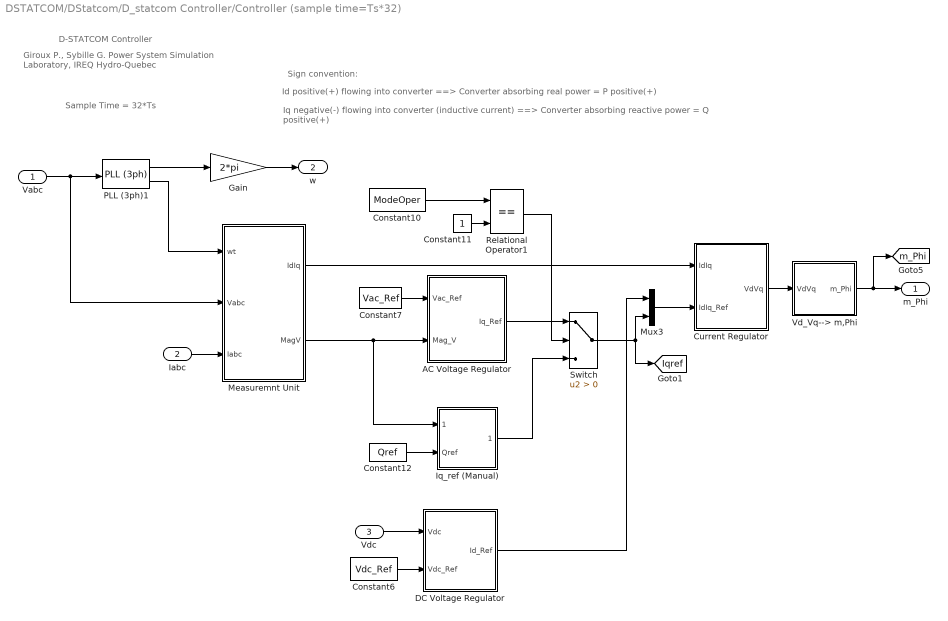
== system DSTATCOM/DStatcom/D_statcom Controller/Controller (sample time=Ts*32) ==
  note: Sample Time = 32*Ts
  note: Id positive(+) flowing into converter ==> Converter absorbing real power = P positive(+)
  note: Sign convention:
  note: Iq negative(-) flowing into converter (inductive current) ==> Converter absorbing reactive power = Q positive(+)
  note: Giroux P., Sybille G.
      | Power System Simulation Laboratory, IREQ
      | Hydro-Quebec
  note: D-STATCOM Controller
  Vabc : Inport  PortDimensions=3
  Iabc : Inport  Port=2  PortDimensions=3
  Vdc : Inport  Port=3  PortDimensions=1
  AC Voltage Regulator : Subsystem  mask(DC Voltage regulator){Kp=Kp_Vac, Ki=Ki_Vac, Ts=32*50e-8}
      mask prompts: Kp "Proportional gain (Kp):"; Ki "Integral gain(Ki)"; Ts "Sample time:"
  Constant10 : Constant  Value=ModeOper
  Constant11 : Constant
  Constant12 : Constant  Value=Qref
  Constant6 : Constant  Value=Vdc_Ref
  Constant7 : Constant  Value=Vac_Ref
  Current Regulator : Subsystem  mask(Current Regulators){Kp=.8, Ki=200, Par_Limits=[1 -1], Init=0, Ts=32*50e-8}
      mask prompts: Kp "Proportional gain (Kp):"; Ki "Integral gain (Ki):"; Par_Limits "Output limits: [ Upper   Lower ]"; Init "Output initial value:"; Ts "Sample time:"
      mask help:
      | Sign convention:
      | Id positive(+) flowing into converter ==> Converter absorbing real power = P positive(+)
      | Iq negative(-) flowing into converter (inductive current) ==> Converter absorbing reactive power = Q positive(+)
  DC Voltage Regulator : Subsystem  mask(DC Voltage regulator){Kp=.001, Ki=.15, Ts=32*50e-8}
      mask prompts: Kp "Proportional gain (Kp):"; Ki "Integral gain(Ki)"; Ts "Sample time:"
  Gain : Gain  Gain=2*pi
  Iq_ref (Manual) : Subsystem
  Measuremnt Unit : Subsystem
  Mux3 : Mux  Inputs=2
  PLL (3ph)1 : spsPLL3phLib/PLL (3ph)  Fmin=45  Par_Init=[3.7 60]  ParK=[60 1400 0]  TcD=1.6e-5  MaxRateChangeFreq=10  FilterCutOffFreq=25  Ts=32*50e-8  AGC=off
  Relational Operator1 : RelationalOperator  Operator===
  Switch : Switch  Criteria=u2 > Threshold
  Vd_Vq--> m,Phi : Subsystem
  m_Phi : Outport  VectorParamsAs1DForOutWhenUnconnected=off
  w : Outport  Port=2  VectorParamsAs1DForOutWhenUnconnected=off
  tag scope: Iqref=global, m_Phi=global
  wires:
  Gain/1 -> w/1
  PLL (3ph)1/1 -> Gain/1
  PLL (3ph)1/2 -> Measuremnt Unit/1(wt)
  Vabc/1 -> Measuremnt Unit/2(Vabc), PLL (3ph)1/1
  Constant6/1 -> DC Voltage Regulator/2(Vdc_Ref)
  Vdc/1 -> DC Voltage Regulator/1(Vdc)
  Constant11/1 -> Relational Operator1/2
  Constant10/1 -> Relational Operator1/1
  Constant12/1 -> Iq_ref (Manual)/2(Qref)
  Iabc/1 -> Measuremnt Unit/3(Iabc)
  Measuremnt Unit/2(MagV) -> AC Voltage Regulator/2(Mag_V), Iq_ref (Manual)/1(MagV)
  Constant7/1 -> AC Voltage Regulator/1(Vac_Ref)
  Measuremnt Unit/1(IdIq) -> Current Regulator/1(IdIq)
  AC Voltage Regulator/1(Iq_Ref) -> Switch/1
  Mux3/1 -> Current Regulator/2(IdIq_Ref)
  Switch/1 -> Mux3/2, [Iqref]
  DC Voltage Regulator/1(Id_Ref) -> Mux3/1
  Iq_ref (Manual)/1(Iqref*) -> Switch/3
  Relational Operator1/1 -> Switch/2
  Current Regulator/1(VdVq) -> Vd_Vq--> m,Phi/1(VdVq)
  Vd_Vq--> m,Phi/1(m_Phi) -> m_Phi/1, [m_Phi]

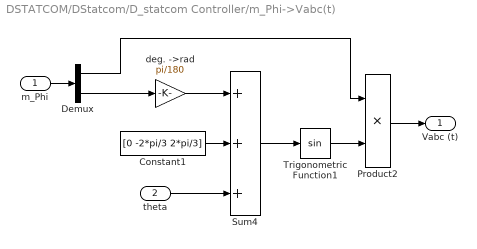
== system DSTATCOM/DStatcom/D_statcom Controller/m_Phi->Vabc(t) ==
  m_Phi : Inport
  theta : Inport  Port=2
  Constant1 : Constant  Value=[0 -2*pi/3 2*pi/3]
  Demux : Demux  Outputs=2
      settings: DisplayOption=none
  Product2 : Product  InputSameDT=on  SaturateOnIntegerOverflow=on  OutDataTypeStr=Inherit: Same as first input
  Sum4 : Sum  Inputs=+++  InputSameDT=on  SaturateOnIntegerOverflow=on  OutDataTypeStr=Inherit: Same as first input
  Trigonometric Function1 : Trigonometry
  deg. ->rad : Gain  Gain=pi/180  SaturateOnIntegerOverflow=on  OutDataTypeStr=Inherit: Same as input  ParamDataTypeStr=Inherit: Same as input
  Vabc (t) : Outport  VectorParamsAs1DForOutWhenUnconnected=off
  wires:
  Trigonometric Function1/1 -> Product2/2
  Sum4/1 -> Trigonometric Function1/1
  Constant1/1 -> Sum4/2
  Demux/1 -> Product2/1
  Product2/1 -> Vabc (t)/1
  m_Phi/1 -> Demux/1
  deg. ->rad/1 -> Sum4/1
  theta/1 -> Sum4/3
  Demux/2 -> deg. ->rad/1

== system DSTATCOM/DStatcom/D_statcom Controller/w->theta ==
  w : Inport
  Constant4 : Constant  Value=2*pi
  Discrete-Time Integrator : DiscreteIntegrator  SampleTime=50e-8  ICPrevOutput=DiscIntNeverNeededParam  ICPrevScaledInput=DiscIntNeverNeededParam
  Math Function : Math  Operator=mod  SignedPower=on
  theta : Outport  VectorParamsAs1DForOutWhenUnconnected=off
  wires:
  Math Function/1 -> theta/1
  w/1 -> Discrete-Time Integrator/1
  Constant4/1 -> Math Function/2
  Discrete-Time Integrator/1 -> Math Function/1

== system DSTATCOM/DStatcom/D_statcom Controller/Controller (sample time=Ts*32)/AC Voltage Regulator ==
  Vac_Ref : Inport
  Mag_V : Inport  Port=2
  Discrete PI Controller : slpidlib/PID Controller  Controller=PI  Form=Parallel  TimeDomain=Discrete-time  UseExternalTs=off  SampleTime=50e-8  IntegratorMethod=Forward Euler  FilterMethod=Forward Euler  ControllerParametersSource=internal  P=.55  I=2500  UseKiTs=off  D=0  N=100  UseFilter=on  TunerSelectOption=Frequency Response Based  InitialConditionSource=internal  InitialConditionForIntegrator=0  InitialConditionForFilter=0  DifferentiatorICPrevScaledInput=0  ExternalReset=none  TrackingMode=off  Kt=1  LimitOutput=on  SatLimitsSource=internal  UpperSaturationLimit=1  LowerSaturationLimit=-1  LinearizeAsGain=off  AntiWindupMode=clamping  Kb=1  LimitIntegrator=off  UpperIntegratorSaturationLimit=inf  LowerIntegratorSaturationLimit=-inf  POutMin=[]  POutMax=[]  IOutMin=[]  IOutMax=[]  DOutMin=[]  DOutMax=[]  NOutMin=[]  NOutMax=[]  SumOutMin=[]  SumOutMax=[]  SaturationOutMin=[]  SaturationOutMax=[]  PParamMin=[]  PParamMax=[]  IParamMin=[]  IParamMax=[]  DParamMin=[]  DParamMax=[]  NParamMin=[]  NParamMax=[]  KbParamMin=[]  KbParamMax=[]  KtParamMin=[]  KtParamMax=[]  KbOutMin=[]  KbOutMax=[]  KtOutMin=[]  KtOutMax=[]  IntegratorOutMin=[]  IntegratorOutMax=[]  FilterOutMin=[]  FilterOutMax=[]  SumI1OutMin=[]  SumI1OutMax=[]  SumI2OutMin=[]  SumI2OutMax=[]  SumI3OutMin=[]  SumI3OutMax=[]  SumI4OutMin=[]  SumI4OutMax=[]  SumDOutMin=[]  SumDOutMax=[]  DifferentiatorOutMin=[]  DifferentiatorOutMax=[]  FilterDiffOutCoefMin=[]  FilterDiffOutCoefMax=[]  ReciprocalOutMin=[]  ReciprocalOutMax=[]  SumDenOutMin=[]  SumDenOutMax=[]  SumNumOutMin=[]  SumNumOutMax=[]  DivideOutMin=[]  DivideOutMax=[]  UdiffTsProdOutMin=[]  UdiffTsProdOutMax=[]  NTsProdOutMin=[]  NTsProdOutMax=[]  UintegralTsProdOutMin=[]  UintegralTsProdOutMax=[]  UngainTsProdOutMin=[]  UngainTsProdOutMax=[]  ClampingZeroOutDataTypeStr=Inherit: Inherit via back propagation  ClampingZeroOutMin=[]  ClampingZeroOutMax=[]  FilterDenConstantOutDataTypeStr=Inherit: Inherit via back propagation  FilterDenConstantOutMin=[]  FilterDenConstantOutMax=[]  PCopyOutDataTypeStr=Inherit: Inherit via back propagation  PCopyOutMin=[]  PCopyOutMax=[]  NCopyOutDataTypeStr=Inherit: Inherit via back propagation  NCopyOutMin=[]  NCopyOutMax=[]  IntegratorContinuousStateAttributes=''  IntegratorStateMustResolveToSignalObject=off  IntegratorRTWStateStorageClass=Auto  FilterContinuousStateAttributes=''  FilterStateMustResolveToSignalObject=off  FilterRTWStateStorageClass=Auto  ParallelPVariant=InternalParameters  IdealPVariant=Disabled  IVariant=InternalParameters  DVariant=Disabled  IntegratorVariant=Discrete  SatVariant=Enabled  AWVariant=DiscClampingParallel  PCopyVariant=Disabled  TRVariant=Disabled  FdbkBlocksVariant=Forward  IdealPFdbkVariant=Disabled  SatFdbkVariant=Disabled  DerivativeFilterVariant=Disabled  NVariant=Disabled  NCopyVariant=Disabled_SignalSpec  FilterICVariant=Disabled  IntegratorICVariant=InternalICs  ExternalResetVariant=Disabled  TRSumVariant=Passthrough  SumFdbkVariant=Disabled  SumVariant=Sum_PI  TsampFilterVariant=InternalTs  TsampNgainVariant=Passthrough  TsampIntegralVariant=Disabled_SignalSpec  ExternalSaturationOutDataTypeStr=Inherit: Same as second input
      settings: AttributesFormatString=P = %<P>\nI = %<I>
  Sum : Sum  Inputs=|+-  InputSameDT=on  SaturateOnIntegerOverflow=on  OutDataTypeStr=Inherit: Same as first input
  Iq_Ref : Outport  InitialOutput=0  VectorParamsAs1DForOutWhenUnconnected=off
  wires:
  Discrete PI Controller/1 -> Iq_Ref/1
  Sum/1 -> Discrete PI Controller/1
  Mag_V/1 -> Sum/2
  Vac_Ref/1 -> Sum/1
